simulink model "q_7"  (R2020a)
settings: Solver=VariableStepAuto  StartTime=0.0  StopTime=10.0  RelTol=1e-3
settings Model: Creator=Admin  LastModifiedBy=Admin

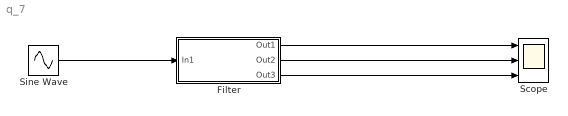
== system q_7 ==
  Filter : Subsystem  TreatAsAtomicUnit=on
  Scope : Scope  NumInputPorts=3
  Sine Wave : Sin  SampleTime=0
  wires:
  Sine Wave/1 -> Filter/1(In1)
  Filter/1(Out1) -> Scope/1
  Filter/2(Out2) -> Scope/2
  Filter/3(Out3) -> Scope/3

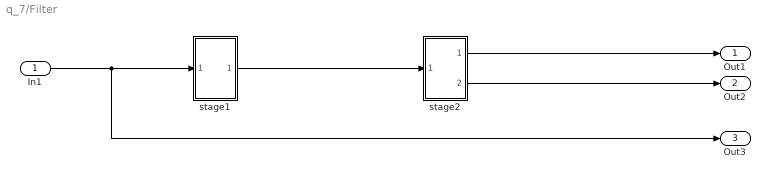
== system q_7/Filter ==
  In1 : Inport
  stage1 : Subsystem
  stage2 : Subsystem
  Out1 : Outport
  Out2 : Outport  Port=2
  Out3 : Outport  Port=3
  wires:
  In1/1 -> Out3/1, stage1/1(In1)
  stage2/1(Out1) -> Out1/1
  stage2/2(Out2) -> Out2/1
  stage1/1(Out1) -> stage2/1(In1)

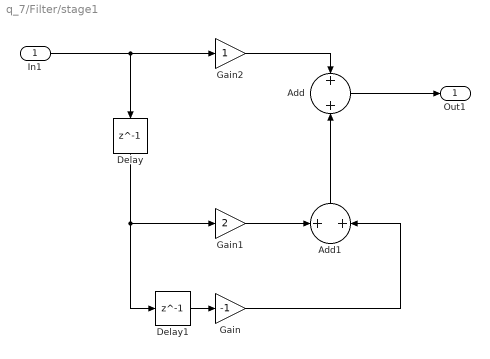
== system q_7/Filter/stage1 ==
  In1 : Inport
  Add : Sum
  Add1 : Sum
  Delay : Delay  DelayLength=1
  Delay1 : Delay  DelayLength=1
  Gain : Gain  Gain=-1
  Gain1 : Gain  Gain=2
  Gain2 : Gain
  Out1 : Outport
  wires:
  In1/1 -> Gain2/1, Delay/1
  Delay/1 -> Delay1/1, Gain1/1
  Gain2/1 -> Add/1
  Add1/1 -> Add/2
  Gain/1 -> Add1/2
  Gain1/1 -> Add1/1
  Add/1 -> Out1/1
  Delay1/1 -> Gain/1

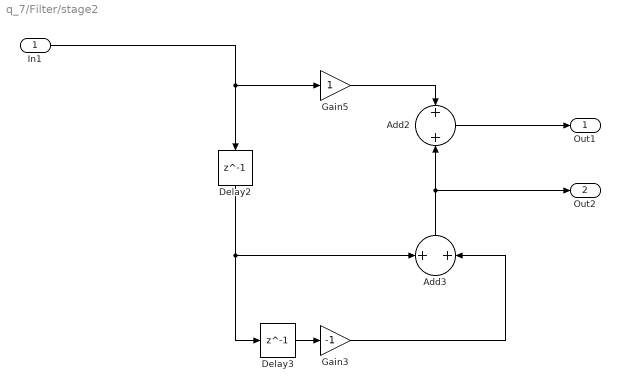
== system q_7/Filter/stage2 ==
  In1 : Inport
  Add2 : Sum
  Add3 : Sum
  Delay2 : Delay  DelayLength=1
  Delay3 : Delay  DelayLength=1
  Gain3 : Gain  Gain=-1
  Gain5 : Gain
  Out1 : Outport
  Out2 : Outport  Port=2
  wires:
  Add3/1 -> Add2/2, Out2/1
  Delay3/1 -> Gain3/1
  In1/1 -> Delay2/1, Gain5/1
  Delay2/1 -> Add3/1, Delay3/1
  Gain5/1 -> Add2/1
  Gain3/1 -> Add3/2
  Add2/1 -> Out1/1
